simulink library "CTRL_SPECCTRL_FB_STRAT1_PREP"  (R2024b)
settings: Solver=VariableStepAuto  StartTime=0.0  StopTime=10.0  RelTol=1e-3
undefined symbols (not defined in the file): p_RadWhlDynFr_m, p_RadWhlDynRe_m, p_RatMotFr_na, p_RatMotRe_na
settings Model: Creator=blatak  LastModifiedBy=blatak

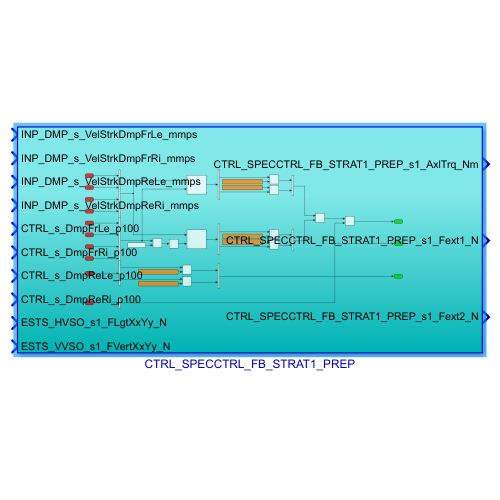
[thumbnail: Simulink's stored preview of the top-level diagram]
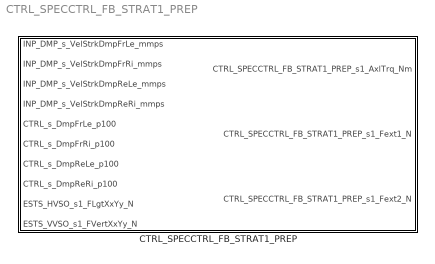
== system CTRL_SPECCTRL_FB_STRAT1_PREP ==
  CTRL_SPECCTRL_FB_STRAT1_PREP : Subsystem

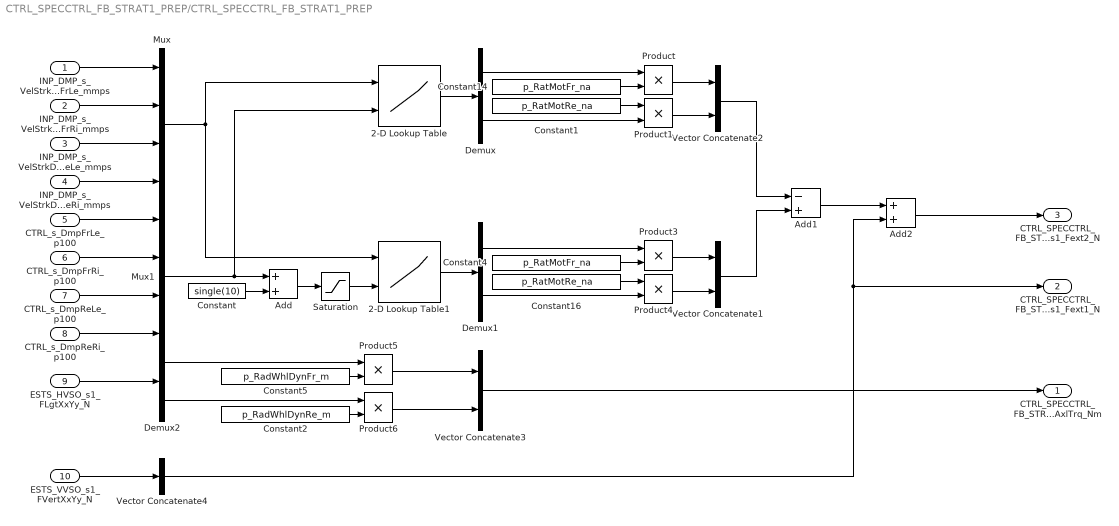
== system CTRL_SPECCTRL_FB_STRAT1_PREP/CTRL_SPECCTRL_FB_STRAT1_PREP ==
  INP_DMP_s_VelStrkDmpFrLe_mmps : Inport
  INP_DMP_s_VelStrkDmpFrRi_mmps : Inport  Port=2
  INP_DMP_s_VelStrkDmpReLe_mmps : Inport  Port=3
  INP_DMP_s_VelStrkDmpReRi_mmps : Inport  Port=4
  CTRL_s_DmpFrLe_p100 : Inport  Port=5
  CTRL_s_DmpFrRi_p100 : Inport  Port=6
  CTRL_s_DmpReLe_p100 : Inport  Port=7
  CTRL_s_DmpReRi_p100 : Inport  Port=8
  ESTS_HVSO_s1_FLgtXxYy_N : Inport  Port=9
  ESTS_VVSO_s1_FVertXxYy_N : Inport  Port=10
  2-D Lookup Table : Lookup_n-D  BreakpointsForDimension1=[1:3]  BreakpointsForDimension2=[1:3]  InternalRulePriority=Speed  RndMeth=Simplest
      settings: InputPortMap=u0,u1
  2-D Lookup Table1 : Lookup_n-D  BreakpointsForDimension1=[1:3]  BreakpointsForDimension2=[1:3]  InternalRulePriority=Speed  RndMeth=Simplest
      settings: InputPortMap=u0,u1
  Add : Sum
  Add1 : Sum  Inputs=-+
  Add2 : Sum
  Constant : Constant  Value=single(10)
  Constant1 : Constant  Value=p_RatMotRe_na
  Constant14 : Constant  Value=p_RatMotFr_na
  Constant16 : Constant  Value=p_RatMotRe_na
  Constant2 : Constant  Value=p_RadWhlDynRe_m
  Constant4 : Constant  Value=p_RatMotFr_na
  Constant5 : Constant  Value=p_RadWhlDynFr_m
  Demux : Demux  Outputs=2
  Demux1 : Demux  Outputs=2
  Demux2 : Demux  Outputs=2
  Mux : Mux
  Mux1 : Mux
  Product{,1,3..6} (6 alike) : Product
  Saturation : Saturate  UpperLimit=100  LowerLimit=0
  Vector Concatenate1 : Concatenate  Mode=Multidimensional array
  Vector Concatenate2 : Concatenate  Mode=Multidimensional array
  Vector Concatenate3 : Concatenate  Mode=Multidimensional array
  Vector Concatenate4 : Concatenate  NumInputs=1  Mode=Multidimensional array
  CTRL_SPECCTRL_FB_STRAT1_PREP_s1_AxlTrq_Nm : Outport
  CTRL_SPECCTRL_FB_STRAT1_PREP_s1_Fext1_N : Outport  Port=2
  CTRL_SPECCTRL_FB_STRAT1_PREP_s1_Fext2_N : Outport  Port=3
  wires:
  Saturation/1 -> 2-D Lookup Table1/2
  2-D Lookup Table1/1 -> Demux1/1
  Add/1 -> Saturation/1
  Add1/1 -> Add2/1
  2-D Lookup Table/1 -> Demux/1
  Product4/1 -> Vector Concatenate1/2
  Product3/1 -> Vector Concatenate1/1
  Constant14/1 -> Product/2
  Product1/1 -> Vector Concatenate2/2
  Constant1/1 -> Product1/1
  Demux2/2 -> Product6/1
  Product5/1 -> Vector Concatenate3/1
  Mux1/1 -> 2-D Lookup Table/2, Add/1
  Demux1/1 -> Product3/1
  Demux1/2 -> Product4/2
  Constant/1 -> Add/2
  Vector Concatenate1/1 -> Add1/2
  Constant4/1 -> Product3/2
  Product/1 -> Vector Concatenate2/1
  Demux/1 -> Product/1
  Mux/1 -> 2-D Lookup Table/1, 2-D Lookup Table1/1
  Vector Concatenate2/1 -> Add1/1
  Constant5/1 -> Product5/2
  Demux2/1 -> Product5/1
  Constant16/1 -> Product4/1
  Demux/2 -> Product1/2
  INP_DMP_s_VelStrkDmpFrLe_mmps/1 -> Mux/1
  INP_DMP_s_VelStrkDmpFrRi_mmps/1 -> Mux/2
  INP_DMP_s_VelStrkDmpReLe_mmps/1 -> Mux/3
  INP_DMP_s_VelStrkDmpReRi_mmps/1 -> Mux/4
  CTRL_s_DmpFrLe_p100/1 -> Mux1/1
  CTRL_s_DmpFrRi_p100/1 -> Mux1/2
  CTRL_s_DmpReLe_p100/1 -> Mux1/3
  CTRL_s_DmpReRi_p100/1 -> Mux1/4
  ESTS_HVSO_s1_FLgtXxYy_N/1 -> Demux2/1
  Product6/1 -> Vector Concatenate3/2
  Constant2/1 -> Product6/2
  Vector Concatenate3/1 -> CTRL_SPECCTRL_FB_STRAT1_PREP_s1_AxlTrq_Nm/1
  ESTS_VVSO_s1_FVertXxYy_N/1 -> Vector Concatenate4/1
  Vector Concatenate4/1 -> CTRL_SPECCTRL_FB_STRAT1_PREP_s1_Fext1_N/1, Add2/2
  Add2/1 -> CTRL_SPECCTRL_FB_STRAT1_PREP_s1_Fext2_N/1
